simulink model "Tarea_Ejercicio10_03_04_17"  (R2013a)
settings: Solver=ode45  SolverMode=SingleTasking  StartTime=0.0  StopTime=10.0  RelTol=1e-3
libraries: powerlib x21, powerlib_meascontrol x4
settings Model: Creator=Juan José  LastModifiedBy=Miguel
settings DataIOCC: SignalLoggingSaveFormat=ModelDataLogs
settings OptimizationCC: BlockReduction=off  BooleanDataType=off
settings DebuggingCC: SaveWithParameterizedLinksMsg=none  SignalResolutionControl=TryResolveAllWithWarning  SolverPrmCheckMsg=none  MultiTaskDSMMsg=warning  MultiTaskCondExecSysMsg=none  StrictBusMsg=None
settings HardwareCC: TargetUnknown=on
settings RTWCC: IncludeERTFirstTime=on

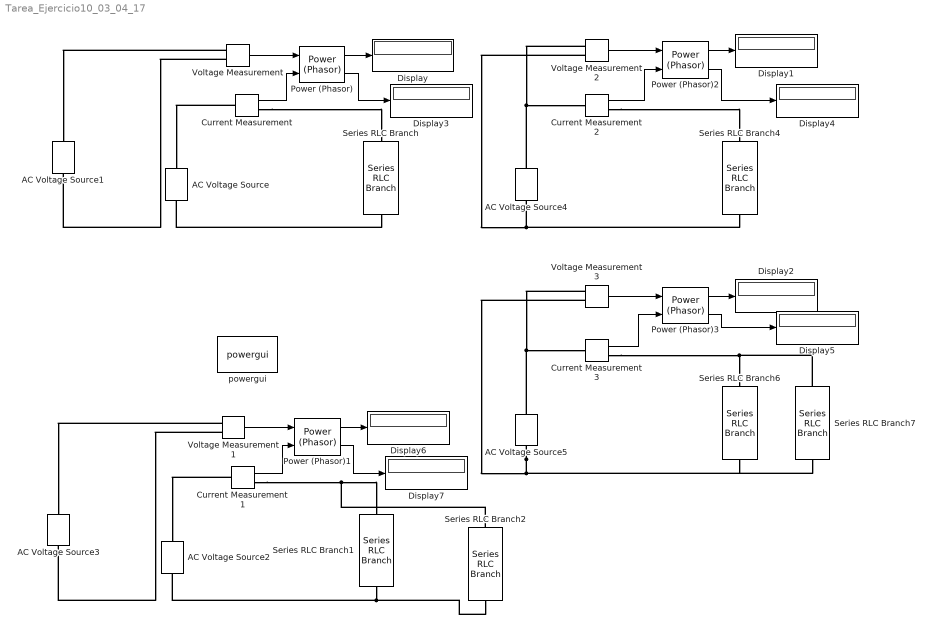
== system Tarea_Ejercicio10_03_04_17 ==
  AC Voltage Source{,2,4..5} (4 alike) : powerlib/Electrical Sources/AC Voltage Source  Amplitude=220*sqrt(2)  Phase=-90  Frequency=60  SampleTime=0  Measurements=None
  AC Voltage Source1 : powerlib/Electrical Sources/AC Voltage Source  Amplitude=125*sqrt(2)  Phase=0  Frequency=60  SampleTime=0  Measurements=None
  AC Voltage Source3 : powerlib/Electrical Sources/AC Voltage Source  Amplitude=125*sqrt(2)  Phase=0  Frequency=60  SampleTime=0  Measurements=None
  Current Measurement{,1..3} (4 alike) : powerlib/Measurements/Current Measurement  PhasorSimulation=on  OutputType=Complex  PSBequivalent=0
  Display{,1..7} (8 alike) : Display
  Power (Phasor){,1..3} (4 alike) : powerlib_meascontrol/Measurements/Power (Phasor)
  Series RLC Branch{,1,4,6} (4 alike) : powerlib/Elements/Series RLC Branch  LConnTagsString=__new0  RConnTagsString=__new0  BranchType=RL  Resistance=4  Inductance=3/(2*pi*60)  SetiL0=off  InitialCurrent=0  Capacitance=1e-6  Setx0=off  InitialVoltage=0  Measurements=None
  Series RLC Branch2 : powerlib/Elements/Series RLC Branch  LConnTagsString=__new0  RConnTagsString=__new0  BranchType=RC  Resistance=1  Inductance=0  SetiL0=off  InitialCurrent=0  Capacitance=1/(8*2*pi*60)  Setx0=off  InitialVoltage=0  Measurements=None
  Series RLC Branch7 : powerlib/Elements/Series RLC Branch  LConnTagsString=__new0  RConnTagsString=__new0  BranchType=RC  Resistance=1  Inductance=0  SetiL0=off  InitialCurrent=0  Capacitance=8/((2*pi*60))  Setx0=off  InitialVoltage=0  Measurements=None
  Voltage Measurement{,1..3} (4 alike) : powerlib/Measurements/Voltage Measurement  PhasorSimulation=on  OutputType=Complex  PSBequivalent=0
  powergui : powerlib/powergui  Priority=1  SimulationMode=Phasor  SolverType=Tustin  SampleTime=50e-6  frequency=60  SPID=off  DisableSnubberDevices=off  DisableRonSwitches=off  DisableVfSwitches=off  SwTol=0  Interpol=off  DisplayEquations=off  frequencyindice=60  Pbase=100e6  ErrMax=1e-4  Iterations=50  UnitsV=kV  UnitsW=MW  FunctionMessages=off  echomessages=off  HookPort=off  EnableUseOfTLC=off  x0status=blocks  RestoreLinks=warning  ResistiveCurrentMeasurement=off  Frange=[0:2:500]  Ylog=off  Xlog=on  ShowGrid=off  save=off  variable=ZData  structure=0  ZoomFFT=off  StartTime=0.0  cycles=1  DisplayStyle=1  fundamental=60  FreqAxis=off  MaxFrequency=1000  frequencyindicesteady=1  RmsSteady=1  display=off  Ts=100  methode=off
  wires:
  Voltage Measurement/1 -> Power (Phasor)/1
  Current Measurement/1 -> Power (Phasor)/2
  Power (Phasor)/1 -> Display/1
  Voltage Measurement2/1 -> Power (Phasor)2/1
  Current Measurement2/1 -> Power (Phasor)2/2
  Power (Phasor)2/1 -> Display1/1
  Voltage Measurement3/1 -> Power (Phasor)3/1
  Current Measurement3/1 -> Power (Phasor)3/2
  Power (Phasor)3/1 -> Display2/1
  Power (Phasor)/2 -> Display3/1
  Power (Phasor)2/2 -> Display4/1
  Power (Phasor)3/2 -> Display5/1
  Voltage Measurement1/1 -> Power (Phasor)1/1
  Current Measurement1/1 -> Power (Phasor)1/2
  Power (Phasor)1/1 -> Display6/1
  Power (Phasor)1/2 -> Display7/1
  connections:
  Series RLC Branch/RConn1 -- AC Voltage Source/LConn1
  Voltage Measurement/LConn1 -- AC Voltage Source1/RConn1
  Voltage Measurement/LConn2 -- AC Voltage Source1/LConn1
  Series RLC Branch4/RConn1 -- Voltage Measurement2/LConn2 -- AC Voltage Source4/LConn1
  Current Measurement2/RConn1 -- Series RLC Branch4/LConn1
  AC Voltage Source4/RConn1 -- Voltage Measurement2/LConn1 -- Current Measurement2/LConn1
  AC Voltage Source5/LConn1 -- Voltage Measurement3/LConn2 -- Series RLC Branch7/RConn1 -- Series RLC Branch6/RConn1
  AC Voltage Source5/RConn1 -- Voltage Measurement3/LConn1 -- Current Measurement3/LConn1
  Current Measurement3/RConn1 -- Series RLC Branch7/LConn1 -- Series RLC Branch6/LConn1
  Current Measurement/LConn1 -- AC Voltage Source/RConn1
  Current Measurement/RConn1 -- Series RLC Branch/LConn1
  Series RLC Branch1/RConn1 -- AC Voltage Source2/LConn1 -- Series RLC Branch2/RConn1
  Voltage Measurement1/LConn2 -- AC Voltage Source3/LConn1
  Current Measurement1/RConn1 -- Series RLC Branch2/LConn1 -- Series RLC Branch1/LConn1
  Voltage Measurement1/LConn1 -- AC Voltage Source3/RConn1
  Current Measurement1/LConn1 -- AC Voltage Source2/RConn1
